simulink model "Torque_Mode_OpenLoop"  (R2014a)
settings: Solver=ode5  StartTime=0.0  StopTime=T_f+0.1  FixedStep=0.001  RelTol=1e-3
InitFcn:
  | load('New_Demo')
  | T_f=37;
undefined symbols (not defined in the file or in its folder): Standard_Devices, UDP_Protocol
libraries: simulink x4, rtwinlib x3, slrtlib x1
(part 2 of 2)

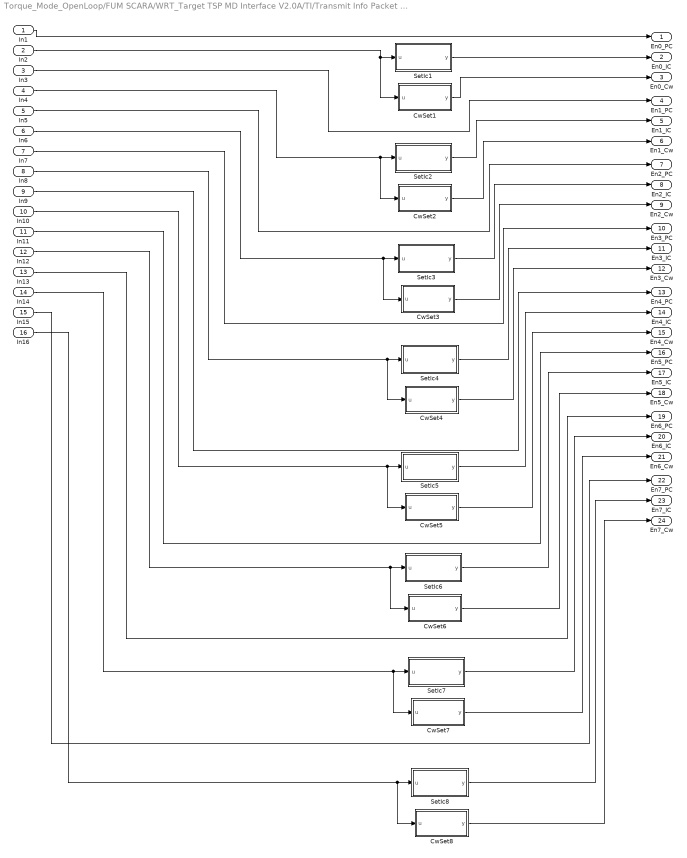
== system Torque_Mode_OpenLoop/FUM SCARA/WRT_Target TSP MD Interface V2.0A/TI/Transmit Info Packet Extract/SetIC ==
  In1 : Inport
  In2 : Inport  Port=2
  In3 : Inport  Port=3
  In4 : Inport  Port=4
  In5 : Inport  Port=5
  In6 : Inport  Port=6
  In7 : Inport  Port=7
  In8 : Inport  Port=8
  In9 : Inport  Port=9
  In10 : Inport  Port=10
  In11 : Inport  Port=11
  In12 : Inport  Port=12
  In13 : Inport  Port=13
  In14 : Inport  Port=14
  In15 : Inport  Port=15
  In16 : Inport  Port=16
  CwSet1 : MATLAB Function  TreatAsAtomicUnit=on
  CwSet2 : MATLAB Function  TreatAsAtomicUnit=on
  CwSet3 : MATLAB Function  TreatAsAtomicUnit=on
  CwSet4 : MATLAB Function  TreatAsAtomicUnit=on
  CwSet5 : MATLAB Function  TreatAsAtomicUnit=on
  CwSet6 : MATLAB Function  TreatAsAtomicUnit=on
  CwSet7 : MATLAB Function  TreatAsAtomicUnit=on
  CwSet8 : MATLAB Function  TreatAsAtomicUnit=on
  SetIc1 : MATLAB Function  TreatAsAtomicUnit=on
  SetIc2 : MATLAB Function  TreatAsAtomicUnit=on
  SetIc3 : MATLAB Function  TreatAsAtomicUnit=on
  SetIc4 : MATLAB Function  TreatAsAtomicUnit=on
  SetIc5 : MATLAB Function  TreatAsAtomicUnit=on
  SetIc6 : MATLAB Function  TreatAsAtomicUnit=on
  SetIc7 : MATLAB Function  TreatAsAtomicUnit=on
  SetIc8 : MATLAB Function  TreatAsAtomicUnit=on
  En0_PC : Outport
  En0_IC : Outport  Port=2
  En0_Cw : Outport  Port=3
  En1_PC : Outport  Port=4
  En1_IC : Outport  Port=5
  En1_Cw : Outport  Port=6
  En2_PC : Outport  Port=7
  En2_IC : Outport  Port=8
  En2_Cw : Outport  Port=9
  En3_PC : Outport  Port=10
  En3_IC : Outport  Port=11
  En3_Cw : Outport  Port=12
  En4_PC : Outport  Port=13
  En4_IC : Outport  Port=14
  En4_Cw : Outport  Port=15
  En5_PC : Outport  Port=16
  En5_IC : Outport  Port=17
  En5_Cw : Outport  Port=18
  En6_PC : Outport  Port=19
  En6_IC : Outport  Port=20
  En6_Cw : Outport  Port=21
  En7_PC : Outport  Port=22
  En7_IC : Outport  Port=23
  En7_Cw : Outport  Port=24
  wires:
  In2/1 -> CwSet1/1(u), SetIc1/1(u)
  In4/1 -> CwSet2/1(u), SetIc2/1(u)
  In6/1 -> CwSet3/1(u), SetIc3/1(u)
  In8/1 -> CwSet4/1(u), SetIc4/1(u)
  In10/1 -> CwSet5/1(u), SetIc5/1(u)
  In12/1 -> CwSet6/1(u), SetIc6/1(u)
  In14/1 -> CwSet7/1(u), SetIc7/1(u)
  In16/1 -> CwSet8/1(u), SetIc8/1(u)
  In1/1 -> En0_PC/1
  SetIc1/1(y) -> En0_IC/1
  CwSet1/1(y) -> En0_Cw/1
  In3/1 -> En1_PC/1
  SetIc2/1(y) -> En1_IC/1
  CwSet2/1(y) -> En1_Cw/1
  In5/1 -> En2_PC/1
  SetIc3/1(y) -> En2_IC/1
  CwSet3/1(y) -> En2_Cw/1
  In7/1 -> En3_PC/1
  SetIc4/1(y) -> En3_IC/1
  CwSet4/1(y) -> En3_Cw/1
  In9/1 -> En4_PC/1
  SetIc5/1(y) -> En4_IC/1
  CwSet5/1(y) -> En4_Cw/1
  In11/1 -> En5_PC/1
  SetIc6/1(y) -> En5_IC/1
  CwSet6/1(y) -> En5_Cw/1
  In13/1 -> En6_PC/1
  SetIc7/1(y) -> En6_IC/1
  CwSet7/1(y) -> En6_Cw/1
  In15/1 -> En7_PC/1
  SetIc8/1(y) -> En7_IC/1
  CwSet8/1(y) -> En7_Cw/1

== system Torque_Mode_OpenLoop/FUM SCARA/WRT_Target TSP MD Interface V2.0A/TI/Transmit Info Packet Extract/SetADC1/ADCconvert1 ==
  ADC_in : Inport
  ADC Mode : Constant  Value=ADC_Mode  SampleTime=-1
  ADC Range : Constant  Value=ADC_Range  SampleTime=-1
  ADC Range Set1 : MATLAB Function  TreatAsAtomicUnit=on
  ADC_Out : Outport
  wires:
  ADC Range Set1/1(ADC_RangeOut) -> ADC_Out/1
  ADC_in/1 -> ADC Range Set1/1(ADC_in)
  ADC Range/1 -> ADC Range Set1/3(ADC_RangeIn)
  ADC Mode/1 -> ADC Range Set1/2(ADC_ModeIn)

== system Torque_Mode_OpenLoop/FUM SCARA/WRT_Target TSP MD Interface V2.0A/TI/Transmit Info Packet Extract/SetADC1/ADCconvert2 ==
  ADC_in : Inport
  ADC Mode : Constant  Value=ADC_Mode  SampleTime=-1
  ADC Range : Constant  Value=ADC_Range  SampleTime=-1
  ADC Range Set1 : MATLAB Function  TreatAsAtomicUnit=on
  ADC_Out : Outport
  wires:
  ADC Range Set1/1(ADC_RangeOut) -> ADC_Out/1
  ADC_in/1 -> ADC Range Set1/1(ADC_in)
  ADC Range/1 -> ADC Range Set1/3(ADC_RangeIn)
  ADC Mode/1 -> ADC Range Set1/2(ADC_ModeIn)

== system Torque_Mode_OpenLoop/FUM SCARA/WRT_Target TSP MD Interface V2.0A/TI/Transmit Info Packet Extract/SetADC1/ADCconvert3 ==
  ADC_in : Inport
  ADC Mode : Constant  Value=ADC_Mode  SampleTime=-1
  ADC Range : Constant  Value=ADC_Range  SampleTime=-1
  ADC Range Set1 : MATLAB Function  TreatAsAtomicUnit=on
  ADC_Out : Outport
  wires:
  ADC Range Set1/1(ADC_RangeOut) -> ADC_Out/1
  ADC_in/1 -> ADC Range Set1/1(ADC_in)
  ADC Range/1 -> ADC Range Set1/3(ADC_RangeIn)
  ADC Mode/1 -> ADC Range Set1/2(ADC_ModeIn)

== system Torque_Mode_OpenLoop/FUM SCARA/WRT_Target TSP MD Interface V2.0A/TI/Transmit Info Packet Extract/SetADC1/ADCconvert4 ==
  ADC_in : Inport
  ADC Mode : Constant  Value=ADC_Mode  SampleTime=-1
  ADC Range : Constant  Value=ADC_Range  SampleTime=-1
  ADC Range Set1 : MATLAB Function  TreatAsAtomicUnit=on
  ADC_Out : Outport
  wires:
  ADC Range Set1/1(ADC_RangeOut) -> ADC_Out/1
  ADC_in/1 -> ADC Range Set1/1(ADC_in)
  ADC Range/1 -> ADC Range Set1/3(ADC_RangeIn)
  ADC Mode/1 -> ADC Range Set1/2(ADC_ModeIn)

== system Torque_Mode_OpenLoop/FUM SCARA/WRT_Target TSP MD Interface V2.0A/TI/Transmit Info Packet Extract/SetADC1/ADCconvert5 ==
  ADC_in : Inport
  ADC Mode : Constant  Value=ADC_Mode  SampleTime=-1
  ADC Range : Constant  Value=ADC_Range  SampleTime=-1
  ADC Range Set1 : MATLAB Function  TreatAsAtomicUnit=on
  ADC_Out : Outport
  wires:
  ADC Range Set1/1(ADC_RangeOut) -> ADC_Out/1
  ADC_in/1 -> ADC Range Set1/1(ADC_in)
  ADC Range/1 -> ADC Range Set1/3(ADC_RangeIn)
  ADC Mode/1 -> ADC Range Set1/2(ADC_ModeIn)

== system Torque_Mode_OpenLoop/FUM SCARA/WRT_Target TSP MD Interface V2.0A/TI/Transmit Info Packet Extract/SetADC1/ADCconvert6 ==
  ADC_in : Inport
  ADC Mode : Constant  Value=ADC_Mode  SampleTime=-1
  ADC Range : Constant  Value=ADC_Range  SampleTime=-1
  ADC Range Set1 : MATLAB Function  TreatAsAtomicUnit=on
  ADC_Out : Outport
  wires:
  ADC Range Set1/1(ADC_RangeOut) -> ADC_Out/1
  ADC_in/1 -> ADC Range Set1/1(ADC_in)
  ADC Range/1 -> ADC Range Set1/3(ADC_RangeIn)
  ADC Mode/1 -> ADC Range Set1/2(ADC_ModeIn)

== system Torque_Mode_OpenLoop/FUM SCARA/WRT_Target TSP MD Interface V2.0A/TI/Transmit Info Packet Extract/SetADC1/ADCconvert7 ==
  ADC_in : Inport
  ADC Mode : Constant  Value=ADC_Mode  SampleTime=-1
  ADC Range : Constant  Value=ADC_Range  SampleTime=-1
  ADC Range Set1 : MATLAB Function  TreatAsAtomicUnit=on
  ADC_Out : Outport
  wires:
  ADC Range Set1/1(ADC_RangeOut) -> ADC_Out/1
  ADC_in/1 -> ADC Range Set1/1(ADC_in)
  ADC Range/1 -> ADC Range Set1/3(ADC_RangeIn)
  ADC Mode/1 -> ADC Range Set1/2(ADC_ModeIn)

== system Torque_Mode_OpenLoop/FUM SCARA/WRT_Target TSP MD Interface V2.0A/TI/Transmit Info Packet Extract/SetADC1/ADCconvert8 ==
  ADC_in : Inport
  ADC Mode : Constant  Value=ADC_Mode  SampleTime=-1
  ADC Range : Constant  Value=ADC_Range  SampleTime=-1
  ADC Range Set1 : MATLAB Function  TreatAsAtomicUnit=on
  ADC_Out : Outport
  wires:
  ADC Range Set1/1(ADC_RangeOut) -> ADC_Out/1
  ADC_in/1 -> ADC Range Set1/1(ADC_in)
  ADC Range/1 -> ADC Range Set1/3(ADC_RangeIn)
  ADC Mode/1 -> ADC Range Set1/2(ADC_ModeIn)

== matlab function Torque_Mode_OpenLoop/FUM SCARA/WRT_Target TSP MD Interface V2.0A/TI/Transmit Info Packet Extract/SetIC/CwSet1 ==
  data: u input; y output
function y = CwSet(u)


y = and(bitshift(u,-28),1);

== matlab function Torque_Mode_OpenLoop/FUM SCARA/WRT_Target TSP MD Interface V2.0A/RI/DAC Set/MATLAB Function ==
  data: DAC_in input; DACEn input; y output
function y = fcn(DAC_in,DACEn)

if DACEn==1 
    
  y =0;
  
else
    
 y=DAC_in;
 
end

== matlab function Torque_Mode_OpenLoop/FUM SCARA/WRT_Target TSP MD Interface V2.0A/TI/Transmit Info Packet Extract/SetIC/CwSet2 ==
  data: u input; y output
function y = CwSet(u)


y = and(bitshift(u,-28),1);

== matlab function Torque_Mode_OpenLoop/FUM SCARA/WRT_Target TSP MD Interface V2.0A/TI/Transmit Info Packet Extract/SetIC/CwSet3 ==
  data: u input; y output
function y = CwSet(u)


y = and(bitshift(u,-28),1);

== matlab function Torque_Mode_OpenLoop/FUM SCARA/WRT_Target TSP MD Interface V2.0A/TI/Transmit Info Packet Extract/SetIC/CwSet4 ==
  data: u input; y output
function y = CwSet(u)


y = and(bitshift(u,-28),1);

== matlab function Torque_Mode_OpenLoop/FUM SCARA/WRT_Target TSP MD Interface V2.0A/TI/Transmit Info Packet Extract/SetIC/CwSet5 ==
  data: u input; y output
function y = CwSet(u)


y = and(bitshift(u,-28),1);

== matlab function Torque_Mode_OpenLoop/FUM SCARA/WRT_Target TSP MD Interface V2.0A/TI/Transmit Info Packet Extract/SetIC/CwSet6 ==
  data: u input; y output
function y = CwSet(u)


y = and(bitshift(u,-28),1);

== matlab function Torque_Mode_OpenLoop/FUM SCARA/WRT_Target TSP MD Interface V2.0A/TI/Transmit Info Packet Extract/SetIC/CwSet7 ==
  data: u input; y output
function y = CwSet(u)


y = and(bitshift(u,-28),1);

== matlab function Torque_Mode_OpenLoop/FUM SCARA/WRT_Target TSP MD Interface V2.0A/TI/Transmit Info Packet Extract/SetIC/CwSet8 ==
  data: u input; y output
function y = CwSet(u)


y = and(bitshift(u,-28),1);

== matlab function Torque_Mode_OpenLoop/FUM SCARA/WRT_Target TSP MD Interface V2.0A/TI/Transmit Info Packet Extract/SetIC/SetIc1 ==
  data: u input; y output
function y = SetIC(u)


y = and(u,16777215);

== matlab function Torque_Mode_OpenLoop/FUM SCARA/WRT_Target TSP MD Interface V2.0A/TI/Transmit Info Packet Extract/SetIC/SetIc2 ==
  data: u input; y output
function y = SetIC(u)


y = and(u,16777215);

== matlab function Torque_Mode_OpenLoop/FUM SCARA/WRT_Target TSP MD Interface V2.0A/TI/Transmit Info Packet Extract/SetIC/SetIc3 ==
  data: u input; y output
function y = SetIC(u)


y = and(u,16777215);

== matlab function Torque_Mode_OpenLoop/FUM SCARA/WRT_Target TSP MD Interface V2.0A/TI/Transmit Info Packet Extract/SetIC/SetIc4 ==
  data: u input; y output
function y = SetIC(u)


y = and(u,16777215);

== matlab function Torque_Mode_OpenLoop/FUM SCARA/WRT_Target TSP MD Interface V2.0A/TI/Transmit Info Packet Extract/SetIC/SetIc5 ==
  data: u input; y output
function y = SetIC(u)


y = and(u,16777215);

== matlab function Torque_Mode_OpenLoop/FUM SCARA/WRT_Target TSP MD Interface V2.0A/TI/Transmit Info Packet Extract/SetIC/SetIc6 ==
  data: u input; y output
function y = SetIC(u)


y = and(u,16777215);

== matlab function Torque_Mode_OpenLoop/FUM SCARA/WRT_Target TSP MD Interface V2.0A/TI/Transmit Info Packet Extract/SetIC/SetIc7 ==
  data: u input; y output
function y = SetIC(u)


y = and(u,16777215);

== stateflow chart Torque_Mode_OpenLoop/FUM SCARA/WRT_Target TSP MD Interface V2.0A/TSP MDI Controller/TSP MDI Control State ==
  state F
    StartStopSetting = 0;
    RstBoard=0;
    ProcessEn=0;
    StartStopEn=0;
  state E
    StartStopSetting = 0;
    RstBoard=1;
    ProcessEn=1;
    StartStopEn=0;
  state D
    StartStopSetting = 0;
    RstBoard=0;
    ProcessEn=0;
    StartStopEn=1;
  state A
    StartStopSetting = 1;
    RstBoard=0;
    ProcessEn=0;
    StartStopEn=1;
  state C
    StartStopSetting = 0;
    RstBoard=0;
    ProcessEn=1;
    StartStopEn=0;
  state B
    StartStopSetting = 0;
    RstBoard=1;
    ProcessEn=1;
    StartStopEn=0;
  E -> F : [hasChangedFrom(CounterIn,MaxCounter)]
  (default) -> A
  D -> E : [hasChangedFrom(CounterIn,MaxCounter-1)]
  A -> B : [hasChangedFrom(CounterIn,0)]
  C -> D : [hasChangedFrom(CounterIn,MaxCounter-2)]
  B -> C : [hasChangedFrom(CounterIn,1)]
  data: CounterIn input double; StartStopEn output double; RstBoard output double; MaxCounter input double; ProcessEn output double; StartStopSetting output double

== matlab function Torque_Mode_OpenLoop/FUM SCARA/WRT_Target TSP MD Interface V2.0A/RI/Byte Gen/MATLAB Function ==
  data: en0_en input; y1 output; en0_rst input; en1_en input; en1_rst input; en2_en input; en2_rst input; en3_en input; en3_rst input; en4_en input; en4_rst input; en5_en input; en5_rst input; en6_en input; en6_rst input; en7_en input; en7_rst input; y2 output
function [y1,y2] = ByteGen(en0_en,en0_rst,en1_en,en1_rst,en2_en,en2_rst,en3_en,en3_rst,en4_en,en4_rst,en5_en,en5_rst,en6_en,en6_rst,en7_en,en7_rst)
y1=en0_en+bitshift(en0_rst,1)+bitshift(en1_en,2)+bitshift(en1_rst,3)+bitshift(en2_en,4)+bitshift(en2_rst,5)+bitshift(en3_en,6)+bitshift(en3_rst,7);
y2=en4_en+bitshift(en4_rst,1)+bitshift(en5_en,2)+bitshift(en5_rst,3)+bitshift(en6_en,4)+bitshift(en6_rst,5)+bitshift(en7_en,6)+bitshift(en7_rst,7);

== matlab function Torque_Mode_OpenLoop/FUM SCARA/WRT_Target TSP MD Interface V2.0A/RI/DAC Set/MATLAB Function1 ==
  data: DAC_in input; DACEn input; y output
function y = fcn(DAC_in,DACEn)

if DACEn==1 
    
  y =0;
  
else
    
 y=DAC_in;
 
end

== matlab function Torque_Mode_OpenLoop/FUM SCARA/WRT_Target TSP MD Interface V2.0A/RI/DAC Set/MATLAB Function2 ==
  data: DAC_in input; DACEn input; y output
function y = fcn(DAC_in,DACEn)

if DACEn==1 
    
  y =0;
  
else
    
 y=DAC_in;
 
end

== matlab function Torque_Mode_OpenLoop/FUM SCARA/WRT_Target TSP MD Interface V2.0A/RI/DAC Set/MATLAB Function3 ==
  data: DAC_in input; DACEn input; y output
function y = fcn(DAC_in,DACEn)

if DACEn==1 
    
  y =0;
  
else
    
 y=DAC_in;
 
end

== matlab function Torque_Mode_OpenLoop/FUM SCARA/WRT_Target TSP MD Interface V2.0A/RI/DAC Set/MATLAB Function4 ==
  data: DAC_in input; DACEn input; y output
function y = fcn(DAC_in,DACEn)

if DACEn==1 
    
  y =0;
  
else
    
 y=DAC_in;
 
end

== matlab function Torque_Mode_OpenLoop/FUM SCARA/WRT_Target TSP MD Interface V2.0A/RI/DAC Set/MATLAB Function5 ==
  data: DAC_in input; DACEn input; y output
function y = fcn(DAC_in,DACEn)

if DACEn==1 
    
  y =0;
  
else
    
 y=DAC_in;
 
end

== matlab function Torque_Mode_OpenLoop/FUM SCARA/WRT_Target TSP MD Interface V2.0A/RI/DAC Set/MATLAB Function6 ==
  data: DAC_in input; DACEn input; y output
function y = fcn(DAC_in,DACEn)

if DACEn==1
    
  y =0;
  
else
    
 y=DAC_in;
 
end

== matlab function Torque_Mode_OpenLoop/FUM SCARA/WRT_Target TSP MD Interface V2.0A/RI/DAC Set/MATLAB Function7 ==
  data: DAC_in input; DACEn input; y output
function y = fcn(DAC_in,DACEn)

if DACEn==1 
    
  y =0;
  
else
    
 y=DAC_in;
 
end

== matlab function Torque_Mode_OpenLoop/MATLAB Function ==
  data: t input; y output; T_f parameter
function y = fcn(t,T_f)
%#codegen
% y =0;   vaccum off and servo off
% y = 15; vaccum off and servo on
% y = 31; vaccum on and servo on

    y = 31; 
    if (t>T_f-0.1)
        y = 0;
     end
end

== matlab function Torque_Mode_OpenLoop/Subsystem/MATLAB Function1 ==
  data: time input; theta1 output; theta2 output; theta1_dt output; theta2_dt output; theta1_ddt output; theta2_ddt output
function [theta1, theta2, theta1_dt, theta2_dt, theta1_ddt, theta2_ddt]  = fcn(time)


time=time*5;
theta1=  (1/4)*(1-cos(time*pi/10));
theta2= (pi/8)*(1-cos(time*pi/10));

theta1_dt= (pi/40)*sin(time*pi/10);
theta2_dt=(pi^2/80)*sin(time*pi/10);

theta1_ddt= (pi^2/400)*cos(time*pi/10);
theta2_ddt=(pi^3/800)*cos(time*pi/10);
% 
% theta(1)=theta1;
% theta(2)=theta2;

== matlab function Torque_Mode_OpenLoop/Subsystem/MATLAB Function2 ==
  data: K input; theta_dd_ref input; Error input; int_Error input; Error_d input; theta_d input; theta input; tau output
function tau = Controller(K,theta_dd_ref,Error,int_Error, Error_d,theta_d,theta)

q2 = theta(2);
qd1 = theta_d(1);
qd2 = theta_d(2);

a1 = 0.4;
x2 = 0.2;

B1 = 3.974;
B2 = 1.771;
B = [B1,0;0,B2];

F1 = 6.657;
F2 = 0.811;
F = [F1,0;0,F2];

Iz1 = 3.307;
Iz2 = 0.083;
m2 = 11.26;

M =[[m2*a1^2 + 2*m2*cos(q2)*a1*x2 + m2*x2^2 + Iz1 + Iz2, m2*x2^2 + a1*m2*cos(q2)*x2 + Iz2]
    [                   m2*x2^2 + a1*m2*cos(q2)*x2 + Iz2,                    m2*x2^2 + Iz2]];

V =[[           -2*a1*m2*qd2*x2*sin(q2),    -a1*m2*qd2*x2*sin(q2)]
    [(a1*m2*x2*sin(q2)*(2*qd1 - qd2))/2, (a1*m2*qd1*x2*sin(q2))/2]];
G = [0;0];

tau1 = M(1,:)*(theta_dd_ref +K(3)*int_Error(1) +K(1)*Error(1)  +K(2)*Error_d(1)) + V(1,:)*theta_d+G(1,:) + B(1,:)*theta_d + F(1,:)*tanh(theta_d);
tau2 = M(2,:)*(theta_dd_ref +K(6)*int_Error(2) +K(4)*Error(2)  +K(5)*Error_d(2)) + V(2,:)*theta_d+G(2,:) + B(2,:)*theta_d + F(2,:)*tanh(theta_d);
% tau1=K(3)*int_Error(1) +K(1)*Error(1)  +K(2)*Error_d(1);
% tau2=K(6)*int_Error(2) +K(4)*Error(2)  +K(5)*Error_d(2);
tau=[tau1;tau2];

== matlab function Torque_Mode_OpenLoop/FUM SCARA/WRT_Target TSP MD Interface V2.0A/TI/Transmit Info Packet Extract/SetIC/SetIc8 ==
  data: u input; y output
function y = SetIC(u)


y = and(u,16777215);

== matlab function Torque_Mode_OpenLoop/FUM SCARA/WRT_Target TSP MD Interface V2.0A/TI/Transmit Info Packet Extract/SetADC1/ADCconvert1/ADC Range Set1 ==
  data: ADC_in input; ADC_ModeIn input; ADC_RangeIn input; ADC_RangeOut output
function ADC_RangeOut = ADC_Range_Set(ADC_in,ADC_ModeIn,ADC_RangeIn)
    
%     Data_out=0.0;
   
    if ADC_in >0
      Data_out=  ADC_in/4095;
    else
     Data_out=   ADC_in/4096;
    end;
    
    switch (ADC_RangeIn)
        case 2
            Data_out= Data_out*5;
        case 3
             Data_out= Data_out*2.5;
        case 4
             Data_out= Data_out*5;
             if ADC_ModeIn ~= 3 
                 Data_out= Data_out+5;
             end;
        otherwise
            Data_out= Data_out*10;
    end;

    if ADC_ModeIn ==3
        Data_out= Data_out*2;
    end ;
    ADC_RangeOut=Data_out;
end

== matlab function Torque_Mode_OpenLoop/FUM SCARA/WRT_Target TSP MD Interface V2.0A/MDI_Setting/MATLAB Function ==
  data: ADC_Mode input; ModeRange output; ADC_Range input
function ModeRange = ByteGen(ADC_Mode,ADC_Range)

ModeRange = ADC_Mode+bitshift( ADC_Range,4);

== matlab function Torque_Mode_OpenLoop/FUM SCARA/WRT_Target TSP MD Interface V2.0A/TI/Transmit Info Packet Extract/SetADC1/ADCconvert2/ADC Range Set1 ==
  data: ADC_in input; ADC_ModeIn input; ADC_RangeIn input; ADC_RangeOut output
function ADC_RangeOut = ADC_Range_Set(ADC_in,ADC_ModeIn,ADC_RangeIn)
    
    Data_out=0.0;
   
    if ADC_in >0
      Data_out=  ADC_in/4095;
    else
     Data_out=   ADC_in/4095;
    end;
    
    switch (ADC_RangeIn)
        case 2
            Data_out= Data_out*5;
        case 3
             Data_out= Data_out*2.5;
        case 4
             Data_out= Data_out*5;
             if ADC_ModeIn ~= 2 
                 Data_out= Data_out+5;
             end;
        otherwise
            Data_out= Data_out*10;
    end;

    if ADC_ModeIn ==2
        Data_out= Data_out*2;
    end ;
    ADC_RangeOut=Data_out;
end

== matlab function Torque_Mode_OpenLoop/FUM SCARA/WRT_Target TSP MD Interface V2.0A/TI/Transmit Info Packet Extract/SetADC1/ADCconvert3/ADC Range Set1 ==
  data: ADC_in input; ADC_ModeIn input; ADC_RangeIn input; ADC_RangeOut output
function ADC_RangeOut = ADC_Range_Set(ADC_in,ADC_ModeIn,ADC_RangeIn)
    
    Data_out=0.0;
   
    if ADC_in >0
      Data_out=  ADC_in/4095;
    else
     Data_out=   ADC_in/4095;
    end;
    
    switch (ADC_RangeIn)
        case 2
            Data_out= Data_out*5;
        case 3
             Data_out= Data_out*2.5;
        case 4
             Data_out= Data_out*5;
             if ADC_ModeIn ~= 2 
                 Data_out= Data_out+5;
             end;
        otherwise
            Data_out= Data_out*10;
    end;

    if ADC_ModeIn ==2
        Data_out= Data_out*2;
    end ;
    ADC_RangeOut=Data_out;
end

== matlab function Torque_Mode_OpenLoop/FUM SCARA/WRT_Target TSP MD Interface V2.0A/TI/Transmit Info Packet Extract/SetADC1/ADCconvert4/ADC Range Set1 ==
  data: ADC_in input; ADC_ModeIn input; ADC_RangeIn input; ADC_RangeOut output
function ADC_RangeOut = ADC_Range_Set(ADC_in,ADC_ModeIn,ADC_RangeIn)
    
    Data_out=0.0;
   
    if ADC_in >0
      Data_out=  ADC_in/4095;
    else
     Data_out=   ADC_in/4095;
    end;
    
    switch (ADC_RangeIn)
        case 2
            Data_out= Data_out*5;
        case 3
             Data_out= Data_out*2.5;
        case 4
             Data_out= Data_out*5;
             if ADC_ModeIn ~= 2 
                 Data_out= Data_out+5;
             end;
        otherwise
            Data_out= Data_out*10;
    end;

    if ADC_ModeIn ==2
        Data_out= Data_out*2;
    end ;
    ADC_RangeOut=Data_out;
end

== matlab function Torque_Mode_OpenLoop/FUM SCARA/WRT_Target TSP MD Interface V2.0A/TI/Transmit Info Packet Extract/SetADC1/ADCconvert5/ADC Range Set1 ==
  data: ADC_in input; ADC_ModeIn input; ADC_RangeIn input; ADC_RangeOut output
function ADC_RangeOut = ADC_Range_Set(ADC_in,ADC_ModeIn,ADC_RangeIn)
    
    Data_out=0.0;
   
    if ADC_in >0
      Data_out=  ADC_in/4095;
    else
     Data_out=   ADC_in/4095;
    end;
    
    switch (ADC_RangeIn)
        case 2
            Data_out= Data_out*5;
        case 3
             Data_out= Data_out*2.5;
        case 4
             Data_out= Data_out*5;
             if ADC_ModeIn ~= 2 
                 Data_out= Data_out+5;
             end;
        otherwise
            Data_out= Data_out*10;
    end;

    if ADC_ModeIn ==2
        Data_out= Data_out*2;
    end ;
    ADC_RangeOut=Data_out;
end

== matlab function Torque_Mode_OpenLoop/FUM SCARA/WRT_Target TSP MD Interface V2.0A/TI/Transmit Info Packet Extract/SetADC1/ADCconvert6/ADC Range Set1 ==
  data: ADC_in input; ADC_ModeIn input; ADC_RangeIn input; ADC_RangeOut output
function ADC_RangeOut = ADC_Range_Set(ADC_in,ADC_ModeIn,ADC_RangeIn)
    
    Data_out=0.0;
   
    if ADC_in >0
      Data_out=  ADC_in/4095;
    else
     Data_out=   ADC_in/4095;
    end;
    
    switch (ADC_RangeIn)
        case 2
            Data_out= Data_out*5;
        case 3
             Data_out= Data_out*2.5;
        case 4
             Data_out= Data_out*5;
             if ADC_ModeIn ~= 2 
                 Data_out= Data_out+5;
             end;
        otherwise
            Data_out= Data_out*10;
    end;

    if ADC_ModeIn ==2
        Data_out= Data_out*2;
    end ;
    ADC_RangeOut=Data_out;
end

== matlab function Torque_Mode_OpenLoop/FUM SCARA/WRT_Target TSP MD Interface V2.0A/TI/Transmit Info Packet Extract/SetADC1/ADCconvert7/ADC Range Set1 ==
  data: ADC_in input; ADC_ModeIn input; ADC_RangeIn input; ADC_RangeOut output
function ADC_RangeOut = ADC_Range_Set(ADC_in,ADC_ModeIn,ADC_RangeIn)
    
    Data_out=0.0;
   
    if ADC_in >0
      Data_out=  ADC_in/4095;
    else
     Data_out=   ADC_in/4095;
    end;
    
    switch (ADC_RangeIn)
        case 2
            Data_out= Data_out*5;
        case 3
             Data_out= Data_out*2.5;
        case 4
             Data_out= Data_out*5;
             if ADC_ModeIn ~= 2 
                 Data_out= Data_out+5;
             end;
        otherwise
            Data_out= Data_out*10;
    end;

    if ADC_ModeIn ==2
        Data_out= Data_out*2;
    end ;
    ADC_RangeOut=Data_out;
end

== matlab function Torque_Mode_OpenLoop/FUM SCARA/WRT_Target TSP MD Interface V2.0A/TI/Transmit Info Packet Extract/SetADC1/ADCconvert8/ADC Range Set1 ==
  data: ADC_in input; ADC_ModeIn input; ADC_RangeIn input; ADC_RangeOut output
function ADC_RangeOut = ADC_Range_Set(ADC_in,ADC_ModeIn,ADC_RangeIn)
    
    Data_out=0.0;
   
    if ADC_in >0
      Data_out=  ADC_in/4095;
    else
     Data_out=   ADC_in/4095;
    end;
    
    switch (ADC_RangeIn)
        case 2
            Data_out= Data_out*5;
        case 3
             Data_out= Data_out*2.5;
        case 4
             Data_out= Data_out*5;
             if ADC_ModeIn ~= 2 
                 Data_out= Data_out+5;
             end;
        otherwise
            Data_out= Data_out*10;
    end;

    if ADC_ModeIn ==2
        Data_out= Data_out*2;
    end ;
    ADC_RangeOut=Data_out;
end
